simulink model "untitled1"  (R2022b)
settings: Solver=FixedStepAuto  StartTime=0.0  StopTime=10.0  FixedStep=0.3  RelTol=1e-3
libraries: robotmobilelib x2
settings Model: Creator=seif  LastModifiedBy=seif

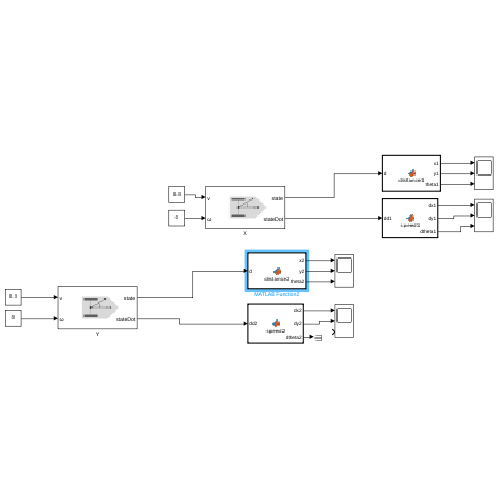
[thumbnail: Simulink's stored preview of the top-level diagram]
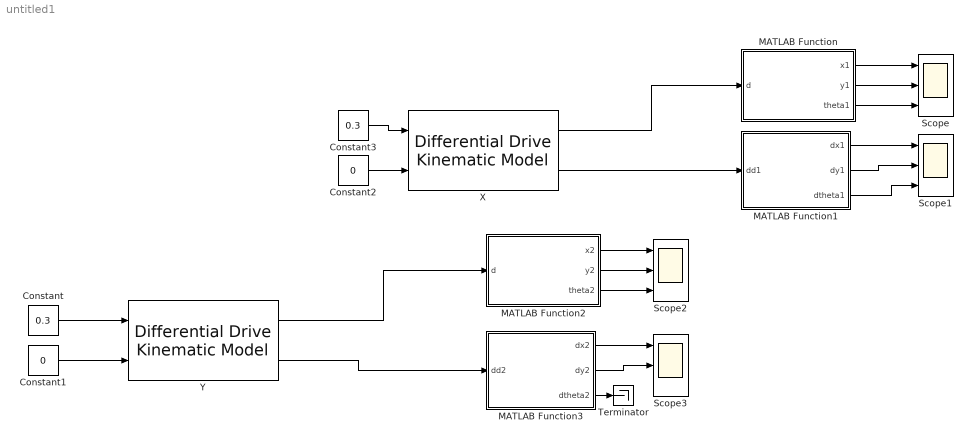
== system untitled1 ==
  Constant : Constant  Value=0.3
  Constant1 : Constant  Value=0
  Constant2 : Constant  Value=0
  Constant3 : Constant  Value=0.3
  MATLAB Function : MATLAB Function  TreatAsAtomicUnit=on
  MATLAB Function1 : MATLAB Function  TreatAsAtomicUnit=on
  MATLAB Function2 : MATLAB Function  TreatAsAtomicUnit=on
  MATLAB Function3 : MATLAB Function  TreatAsAtomicUnit=on
  Scope{,1..3} (4 alike) : Scope  NumInputPorts=3
  Terminator : Terminator
  X : robotmobilelib/Differential Drive Kinematic Model  VehicleInputs=Vehicle Speed & Heading Angular Velocity  WheelRadius=0.05  WheelSpeedRange=[-inf inf]  TrackWidth=0.2  InitialState=[0; 0; 0]  SimulateUsing=Interpreted execution
  Y : robotmobilelib/Differential Drive Kinematic Model  VehicleInputs=Vehicle Speed & Heading Angular Velocity  WheelRadius=0.05  WheelSpeedRange=[-inf inf]  TrackWidth=0.2  InitialState=[0; 0; 0]  SimulateUsing=Interpreted execution
  wires:
  Y/2 -> MATLAB Function3/1(dd2)
  Y/1 -> MATLAB Function2/1(d)
  Constant1/1 -> Y/2
  X/1 -> MATLAB Function/1(d)
  MATLAB Function3/3(dtheta2) -> Terminator/1
  Constant2/1 -> X/2
  X/2 -> MATLAB Function1/1(dd1)
  Constant/1 -> Y/1
  Constant3/1 -> X/1
  MATLAB Function/1(x1) -> Scope/1
  MATLAB Function/2(y1) -> Scope/2
  MATLAB Function/3(theta1) -> Scope/3
  MATLAB Function1/1(dx1) -> Scope1/1
  MATLAB Function1/2(dy1) -> Scope1/2
  MATLAB Function1/3(dtheta1) -> Scope1/3
  MATLAB Function2/1(x2) -> Scope2/1
  MATLAB Function2/2(y2) -> Scope2/2
  MATLAB Function2/3(theta2) -> Scope2/3
  MATLAB Function3/1(dx2) -> Scope3/1
  MATLAB Function3/2(dy2) -> Scope3/2

== matlab function untitled1/MATLAB Function1 ==
  data: dd1 input; dx1 output; dy1 output; dtheta1 output
function [dx1, dy1, dtheta1] = speed1(dd1)
  % Perform some calculations on the input u to compute x, y, and theta
  dx1 = dd1(1);
  dy1 = dd1(2);
  dtheta1 = dd1(3);
  
  % Print the output values using sprintf
%   disp(['dx1 = ', sprintf('%f', dx1)]);
%   disp(['dy1 = ', sprintf('%f', dy1)]);
%   disp(['dtheta1 = ', sprintf('%f', dtheta1)]);
end

== matlab function untitled1/MATLAB Function ==
  settings: updateMethod=DISCRETE
  data: x1 output; y1 output; d input; theta1 output
function [x1, y1, theta1] = distance1(d)
  % Perform some calculations on the input u to compute x, y, and theta
  
  rng('shuffle')
  persistent initialpos;

  if isempty(initialpos)
    initialpos= ((rand()*0.3)+0.85);
  end
  
  x1 = d(1)-initialpos;
  y1 = 0;
  theta1 = d(3);
  
  % Print the output values using sprintf
%   disp(['x1 = ', sprintf('%f', x1)]);
%   disp(['y1 = ', sprintf('%f', y1)]);
%   disp(['theta1 = ', sprintf('%f', theta1)]);
  disp(['init = ', sprintf('%f', initialpos)]);
end

%((rand()*0.3)+0.85)

== matlab function untitled1/MATLAB Function2 ==
  settings: updateMethod=DISCRETE
  data: x2 output; y2 output; d input; theta2 output
function [x2, y2, theta2] = distance2(d)
  % Perform some calculations on the input u to compute x, y, and theta
  rng('shuffle')
  persistent initialpos1;
  if isempty(initialpos1)
    initialpos1 = ((rand()*0.3)+0.85);
  end
  
  x2 = 0;
  y2 = d(1)-initialpos1;
  theta2 = d(3);

  
  % Print the output values using sprintf
%   disp(['x2 = ', sprintf('%f', x2)]);
%   disp(['y2 = ', sprintf('%f', y2)]);
%   disp(['theta2 = ', sprintf('%f', theta2)]);
    disp(['init2= ', sprintf('%f', initialpos1)])
end

== matlab function untitled1/MATLAB Function3 ==
  data: dd2 input; dx2 output; dy2 output; dtheta2 output
function [dx2, dy2, dtheta2] = speed2(dd2)
  % Perform some calculations on the input u to compute x, y, and theta
  dx2 = dd2(1);
  dy2 = dd2(2);
  dtheta2 = dd2(3);
  
  % Print the output values using sprintf
%   disp(['dx2 = ', sprintf('%f', dx2)]);
%   disp(['dy2 = ', sprintf('%f', dy2)]);
%   disp(['dtheta2 = ', sprintf('%f', dtheta2)]);
end
